simulink library "LatTtc"  (Simulink 8.1)
settings: Solver=ode1  StartTime=0.0  StopTime=Inf  FixedStep=0.001  RelTol=1e-3
PostLoadFcn:
  | , if any(exist('dsrtsu_mdlpostloadfcn', 'file') == [2, 3, 6]), try dsrtsu_mdlpostloadfcn('Execute', bdroot); catch fprintf('Error in PostLoadFcn (dsrtsu_mdlpostloadfcn) for model "%s":\n %s\n', bdroot, lasterr); end, end,
undefined symbols (not defined in the file or in its folder): KIFO_TTCDefault_s
libraries: hcu_lib x2
settings Model: DSRTSU_INTERNAL_RTI_VER=450  DSRTSU_INTERNAL_RTI_TYPE=rti1401  RTICANMMDATA=struct('GeneralSetupData',struct('modelroot','D:\PROJECTS\HAITEC\IDIADA_HAITEC_SVN\Phase3\branches\Model_with_Pedestrians\AdasDragon\software\sw_development\arch\app\ifo','generalsettings',struct('filesettings',struct('destfolder',struct('Name','RTICANMM_FILES','Check',1),'buildfolder',struct('Name','.','Check',1),'AbsDestfolder',struct('Name','D:\PROJECTS\HAITEC\IDIADA_HAITEC_SVN\Phase3\branches\Model_with_Pedestrians\AdasDragon\software\sw_development\arch\app\ifo\RTICANMM_FILES'),'AbsBuildfolder',struct('Name','D:\PROJECTS\HAITEC\IDIADA_HAITEC_SVN\Phase3\branches\Model_with_Pedestrians\AdasDragon\software\sw_development\arch\app\ifo'))),'options',struct('addpaths',1,'rmpaths',1,'addtrcexclusion',logical(1),'cannavigator',struct('checkmonitoring',0),'show_usrtrc',0,'use_usrtrc',0),'advanced',struct('options',[1 1 1 1 1 1 1 1 1 1 1 1 1 1 1 1 1 1 1 1 1 1 1 1 1 1 1 1 1 1 1 1 1 1 1 1 1 1 1 1 1 1 1 1 1 1 1 1 1 1 1 1 1 1 1 1 1 1 1 1 1 1 1 1 1 1 1 1 1 1 1 1 1 1 1 1 1 1 1 1 1 1 1 1 1 1 1 1 1 1 1 1 1 1 1 1 1 1 1 1]),'MPSetup',{{}},'modelname','LatTtc','block','LatTtc'))  DSRTSU_INTERNAL_RTIFPGA=40  Creator=tescamilla  LastModifiedBy=tescamilla

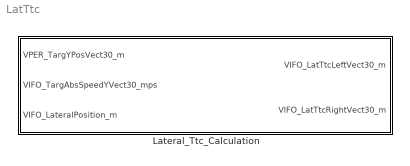
== system LatTtc ==
  Lateral_Ttc_Calculation : Subsystem

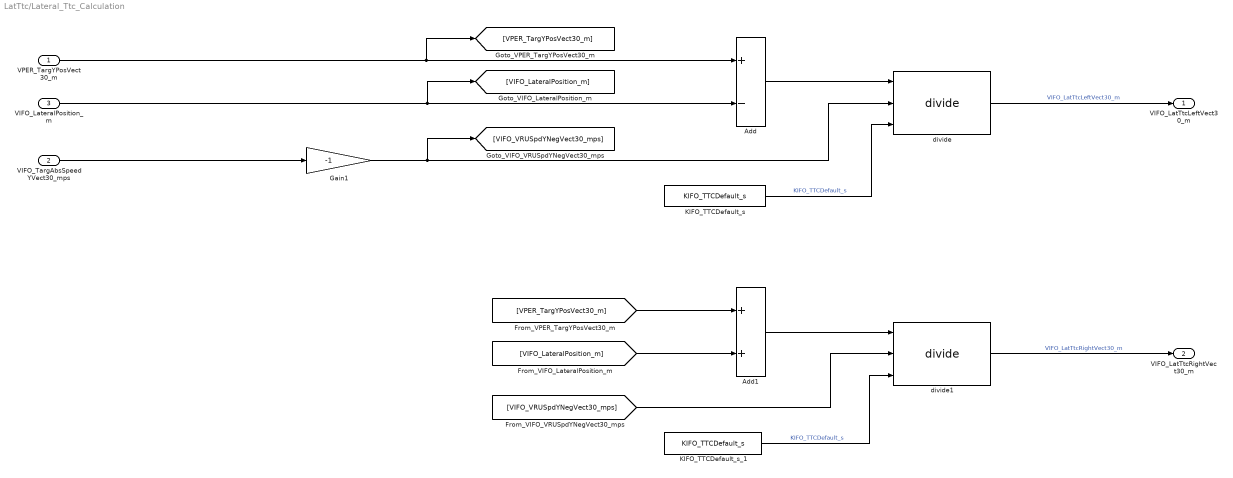
== system LatTtc/Lateral_Ttc_Calculation ==
  VPER_TargYPosVect30_m : Inport
  VIFO_TargAbsSpeedYVect30_mps : Inport  Port=2
  VIFO_LateralPosition_m : Inport  Port=3
  Add : Sum  Inputs=+-
  Add1 : Sum
  Gain1 : Gain  Gain=-1
  KIFO_TTCDefault_s : Constant  Value=KIFO_TTCDefault_s
  KIFO_TTCDefault_s_1 : Constant  Value=KIFO_TTCDefault_s
  divide : hcu_lib/divide
  divide1 : hcu_lib/divide
  VIFO_LatTtcLeftVect30_m : Outport
  VIFO_LatTtcRightVect30_m : Outport  Port=2
  wires:
  VIFO_LateralPosition_m/1 -> Add/2, [VIFO_LateralPosition_m]
  VPER_TargYPosVect30_m/1 -> Add/1, [VPER_TargYPosVect30_m]
  Add/1 -> divide/1
  VIFO_TargAbsSpeedYVect30_mps/1 -> Gain1/1
  Gain1/1 -> divide/2, [VIFO_VRUSpdYNegVect30_mps]
  KIFO_TTCDefault_s/1 -> divide/3  "KIFO_TTCDefault_s"
  divide/1 -> VIFO_LatTtcLeftVect30_m/1  "VIFO_LatTtcLeftVect30_m"
  divide1/1 -> VIFO_LatTtcRightVect30_m/1  "VIFO_LatTtcRightVect30_m"
  [VPER_TargYPosVect30_m] -> Add1/1
  [VIFO_LateralPosition_m] -> Add1/2
  Add1/1 -> divide1/1
  [VIFO_VRUSpdYNegVect30_mps] -> divide1/2
  KIFO_TTCDefault_s_1/1 -> divide1/3  "KIFO_TTCDefault_s"
